simulink model "sim_tcst_2024_att_ctrl"  (R2020a)
settings: Solver=ode4  StartTime=0.0  StopTime=30.0  FixedStep=0.01  RelTol=1e-3
values from neighbouring files (symbols this model uses):
  beta0 = 2    [init_tcst_2024_att_ctrl.m]
  c1_diff_sigma_bar_w = diag([12; 12; 12])    [init_tcst_2024_att_ctrl.m]
  c1_diff_ui = diag([25; 30; 20])    [init_tcst_2024_att_ctrl.m]
  c2_diff_sigma_bar_w = diag([12; 12; 12])    [init_tcst_2024_att_ctrl.m]
  c2_diff_ui = diag([50; 50; 10])    [init_tcst_2024_att_ctrl.m]
  c3_diff_sigma_bar_w = diag([15; 15; 15])    [init_tcst_2024_att_ctrl.m]
  c3_diff_ui = diag([15; 15; 10])    [init_tcst_2024_att_ctrl.m]
  dw_aa_t = 0.2 * ones(3, 5) + ( 1.0 - 0.2 ) * rand(3, 5)    [init_tcst_2024_att_ctrl.m]
  dw_ff_t = [ 0.4 * ones(1, 5) + ( 1.0 - 0.4 ) * rand(1, 5);                      0.4 * ones(1, 5) + ( 1.0 - 0.4 ) * rand(1, 5);                      0.2 * ones(1, 5) + ( 0.6 - 0.2 ) * rand(1, 5) ]    [init_tcst_2024_att_ctrl.m]
  dw_phi_t = ( - pi / 2 ) * ones(3, 5) + ( pi / 2 - ( - pi / 2 ) ) * rand(3, 5)    [init_tcst_2024_att_ctrl.m]
  dwci_init = zeros(3,5)    [init_tcst_2024_att_ctrl.m]
  err_Ri_bar_init = zeros(3,NF)    [init_tcst_2024_att_ctrl.m]
  Fi_init = zeros(3,NF)    [init_tcst_2024_att_ctrl.m]
  h1w = diag([20.0; 20.0; 20.0])    [init_tcst_2024_att_ctrl.m]
  h2w = diag([30.0; 35.0; 35.0])    [init_tcst_2024_att_ctrl.m]
  h3w = diag([30.0; 25.0; 30.0])    [init_tcst_2024_att_ctrl.m]
  Ji = zeros(3,3,NF)    [init_tcst_2024_att_ctrl.m]
  kr1 = 10    [init_tcst_2024_att_ctrl.m]
  kr2 = 10    [init_tcst_2024_att_ctrl.m]
  kr3 = 5    [init_tcst_2024_att_ctrl.m]
  Lamd_diff_sigma_bar_w = 0.8    [init_tcst_2024_att_ctrl.m]
  Lamd_diff_ui = 0.8    [init_tcst_2024_att_ctrl.m]
  mu_d_w = 100    [init_tcst_2024_att_ctrl.m]
  pos0 = zeros(3, 1)    [init_tcst_2024_att_ctrl.m]
  PZ0 = P0(3)    [init_tcst_2024_att_ctrl.m]
  PZ1 = 10    [init_tcst_2024_att_ctrl.m]
  Qci_init = repmat([1;0;0;0],1,NF)    [init_tcst_2024_att_ctrl.m]
  Qei_init = zeros(4,NF)    [init_tcst_2024_att_ctrl.m]
  R0 = 4    [init_tcst_2024_att_ctrl.m]
  R1 = 8    [init_tcst_2024_att_ctrl.m]
  Rci_init = zeros(3,3,NF)    [init_tcst_2024_att_ctrl.m]
  Rei_init = zeros(3,3,NF)    [init_tcst_2024_att_ctrl.m]
  Ri_init = zeros(3,3,NF)    [init_tcst_2024_att_ctrl.m]
  Rx2 = 10    [init_tcst_2024_att_ctrl.m]
  Ry2 = 6    [init_tcst_2024_att_ctrl.m]
  Rz2 = 4    [init_tcst_2024_att_ctrl.m]
  T0 = 0    [init_tcst_2024_att_ctrl.m]
  T1 = tseq1    (= 10)    [init_tcst_2024_att_ctrl.m]
  T2 = tseq1 + tseq12 + tseq2    (= 30)    [init_tcst_2024_att_ctrl.m]
  ui_init = zeros(3,NF)    [init_tcst_2024_att_ctrl.m]
  V_Phi_Rei_init = zeros(3,NF)    [init_tcst_2024_att_ctrl.m]
  vel0 = zeros(3, 1)    [init_tcst_2024_att_ctrl.m]
  wci_init = zeros(3,5)    [init_tcst_2024_att_ctrl.m]
  wei_init = zeros(3,NF)    [init_tcst_2024_att_ctrl.m]
  zeta_diff_sigma_bar_w = 0.3    [init_tcst_2024_att_ctrl.m]
  zeta_diff_ui = 0.05    [init_tcst_2024_att_ctrl.m]
undefined symbols (not defined in the file or in its folder): cal_frac_squ, p_alfaw1, p_alfaw2, q_alfaw1, q_alfaw2, Qi_init, wi_init
(part 2 of 4)

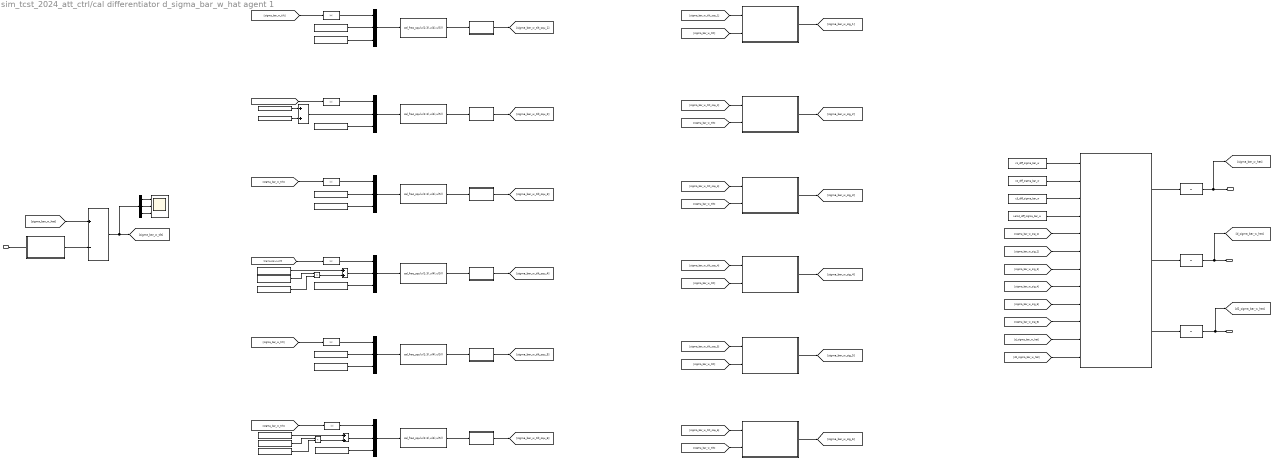
== system sim_tcst_2024_att_ctrl/cal differentiator d_sigma_bar_w_hat agent 1 ==
  x : Inport
  Abs{,1..5} (6 alike) : Abs
  Add : Sum
  Add1 : Sum
  Add2 : Sum
  Add3 : Sum  Inputs=+-
  Constant : Constant  Value=0
  Constant{97,100,105,107,109} (5 alike) : Constant
  Constant{98..99,101,108,110..111} (6 alike) : Constant  Value=3
  Constant102 : Constant  Value=2
  Constant103 : Constant  Value=c1_diff_sigma_bar_w
  Constant104 : Constant  Value=c2_diff_sigma_bar_w
  Constant106 : Constant  Value=c3_diff_sigma_bar_w
  Constant112 : Constant  Value=2
  Constant113 : Constant  Value=Lamd_diff_sigma_bar_w
  Constant161 : Constant  Value=zeta_diff_sigma_bar_w
  Constant162 : Constant  Value=zeta_diff_sigma_bar_w
  Constant163 : Constant  Value=zeta_diff_sigma_bar_w
  Demux2 : Demux  Outputs=3
  Integrator2 : Integrator  InitialCondition=zeros(3,1)
  Integrator3 : Integrator  InitialCondition=zeros(3,1)
  Integrator4 : Integrator  InitialCondition=zeros(3,1)
  Interpreted MATLAB Function{,20..24} (6 alike) : MATLABFcn  MATLABFcn=cal_frac_squ(u(1:3),u(4),u(5))
  Mux{19..24} (6 alike) : Mux  Inputs=3
  Product : Product
  Product1 : Product
  cal differentiator : MATLAB Function  TreatAsAtomicUnit=on
  cal sig : MATLAB Function  TreatAsAtomicUnit=on
  cal sig1 : MATLAB Function  TreatAsAtomicUnit=on
  cal sig2 : MATLAB Function  TreatAsAtomicUnit=on
  cal sig3 : MATLAB Function  TreatAsAtomicUnit=on
  cal sig4 : MATLAB Function  TreatAsAtomicUnit=on
  cal sig5 : MATLAB Function  TreatAsAtomicUnit=on
  choose sigma_bar_w : MATLAB Function  TreatAsAtomicUnit=on
  sigma_bar_w_tilt : Scope  NumInputPorts=3
  trans to column20 : MATLAB Function  TreatAsAtomicUnit=on
  trans to column21 : MATLAB Function  TreatAsAtomicUnit=on
  trans to column22 : MATLAB Function  TreatAsAtomicUnit=on
  trans to column23 : MATLAB Function  TreatAsAtomicUnit=on
  trans to column24 : MATLAB Function  TreatAsAtomicUnit=on
  trans to column25 : MATLAB Function  TreatAsAtomicUnit=on
  Out1 : Outport
  Out2 : Outport  Port=2
  Out3 : Outport  Port=3
  wires:
  Abs/1 -> Mux22/1
  [sigma_bar_w_tilt] -> cal sig/2(y)
  cal sig1/1(z) -> [sigma_bar_w_sig_2]
  [d2_sigma_bar_w_hat] -> cal differentiator/12(d2_sigma_bar_v_hat)
  trans to column23/1(y) -> [sigma_bar_w_tilt_squ_3]
  Add/1 -> Mux21/2
  Demux2/1 -> sigma_bar_w_tilt/1
  [sigma_bar_w_tilt] -> cal sig4/2(y)
  Product1/1 -> Add2/2
  Add2/1 -> Mux19/2
  [d_sigma_bar_w_hat] -> cal differentiator/11("d_sigma_bar_v_hat ")
  [sigma_bar_w_sig_3] -> cal differentiator/7(sigma_bar_v_sig_3)
  trans to column24/1(y) -> [sigma_bar_w_tilt_squ_4]
  Constant107/1 -> Mux21/3
  [sigma_bar_w_sig_5] -> cal differentiator/9(sigma_bar_v_sig_5)
  Constant97/1 -> Mux22/3
  cal sig/1(z) -> [sigma_bar_w_sig_1]
  trans to column22/1(y) -> [sigma_bar_w_tilt_squ_1]
  [sigma_bar_w_tilt_squ_3] -> cal sig2/1(x)
  [sigma_bar_w_tilt] -> Abs3/1
  Interpreted MATLAB Function24/1 -> trans to column25/1(x)
  [sigma_bar_w_sig_1] -> cal differentiator/5(sigma_bar_v_sig_1)
  cal differentiator/1(d_sigma_bar_v_hat) -> Integrator2/1
  Constant110/1 -> Mux24/3
  cal sig5/1(z) -> [sigma_bar_w_sig_5]
  [sigma_bar_w_tilt] -> Abs4/1
  Demux2/3 -> sigma_bar_w_tilt/3
  cal sig2/1(z) -> [sigma_bar_w_sig_3]
  Constant112/1 -> Product/1
  Constant/1 -> Mux22/2
  cal differentiator/3(d_d2sigma_bar_v_hat) -> Integrator4/1
  Abs3/1 -> Mux24/1
  trans to column21/1(y) -> [sigma_bar_w_tilt_squ_2]
  Constant99/1 -> Add2/1
  Constant103/1 -> cal differentiator/1(c1)
  Mux19/1 -> Interpreted MATLAB Function24/1
  [sigma_bar_w_tilt_squ_6] -> cal sig3/1(x)
  Constant106/1 -> cal differentiator/3(c3)
  [sigma_bar_w_tilt] -> Abs2/1
  [sigma_bar_w_tilt_squ_2] -> cal sig1/1(x)
  Constant162/1 -> Product/2
  Product/1 -> Add1/2
  [sigma_bar_w_sig_4] -> cal differentiator/8(sigma_bar_v_sig_4)
  [sigma_bar_w_hat] -> Add3/1
  Constant102/1 -> Mux20/2
  Add3/1 -> Demux2/1, [sigma_bar_w_tilt]
  cal differentiator/2(d_dsigma_bar_v_hat) -> Integrator3/1
  [sigma_bar_w_tilt] -> Abs5/1
  [sigma_bar_w_tilt] -> cal sig2/2(y)
  [sigma_bar_w_sig_6] -> cal differentiator/10(sigma_bar_v_sig_6)
  trans to column20/1(y) -> [sigma_bar_w_tilt_squ_5]
  Constant104/1 -> cal differentiator/2(c2)
  Constant101/1 -> Mux20/3
  Mux22/1 -> Interpreted MATLAB Function/1
  Constant163/1 -> Product1/2
  Abs2/1 -> Mux23/1
  Interpreted MATLAB Function21/1 -> trans to column21/1(x)
  Interpreted MATLAB Function23/1 -> trans to column24/1(x)
  Mux23/1 -> Interpreted MATLAB Function22/1
  cal sig3/1(z) -> [sigma_bar_w_sig_6]
  Abs4/1 -> Mux19/1
  trans to column25/1(y) -> [sigma_bar_w_tilt_squ_6]
  Constant113/1 -> cal differentiator/4(chi_t)
  choose sigma_bar_w/1(y) -> Add3/2
  Interpreted MATLAB Function/1 -> trans to column22/1(x)
  Interpreted MATLAB Function20/1 -> trans to column20/1(x)
  Constant108/1 -> Mux23/3
  [sigma_bar_w_sig_2] -> cal differentiator/6(sigma_bar_v_sig_2)
  [sigma_bar_w_tilt] -> cal sig1/2(y)
  [sigma_bar_w_tilt_squ_1] -> cal sig/1(x)
  Constant100/1 -> Product1/1
  Abs1/1 -> Mux21/1
  Demux2/2 -> sigma_bar_w_tilt/2
  Integrator4/1 -> [d2_sigma_bar_w_hat], Out3/1
  [sigma_bar_w_tilt_squ_4] -> cal sig4/1(x)
  Abs5/1 -> Mux20/1
  Constant98/1 -> Mux19/3
  Constant111/1 -> Add1/1
  [sigma_bar_w_tilt] -> cal sig5/2(y)
  Constant109/1 -> Mux23/2
  [sigma_bar_w_tilt] -> Abs/1
  Mux24/1 -> Interpreted MATLAB Function23/1
  [sigma_bar_w_tilt] -> Abs1/1
  [sigma_bar_w_tilt_squ_5] -> cal sig5/1(x)
  Add1/1 -> Mux24/2
  cal sig4/1(z) -> [sigma_bar_w_sig_4]
  Constant161/1 -> Add/2
  [sigma_bar_w_tilt] -> cal sig3/2(y)
  Mux21/1 -> Interpreted MATLAB Function21/1
  Interpreted MATLAB Function22/1 -> trans to column23/1(x)
  Mux20/1 -> Interpreted MATLAB Function20/1
  x/1 -> choose sigma_bar_w/1(x)
  Constant105/1 -> Add/1
  Integrator2/1 -> [sigma_bar_w_hat], Out1/1
  Integrator3/1 -> [d_sigma_bar_w_hat], Out2/1

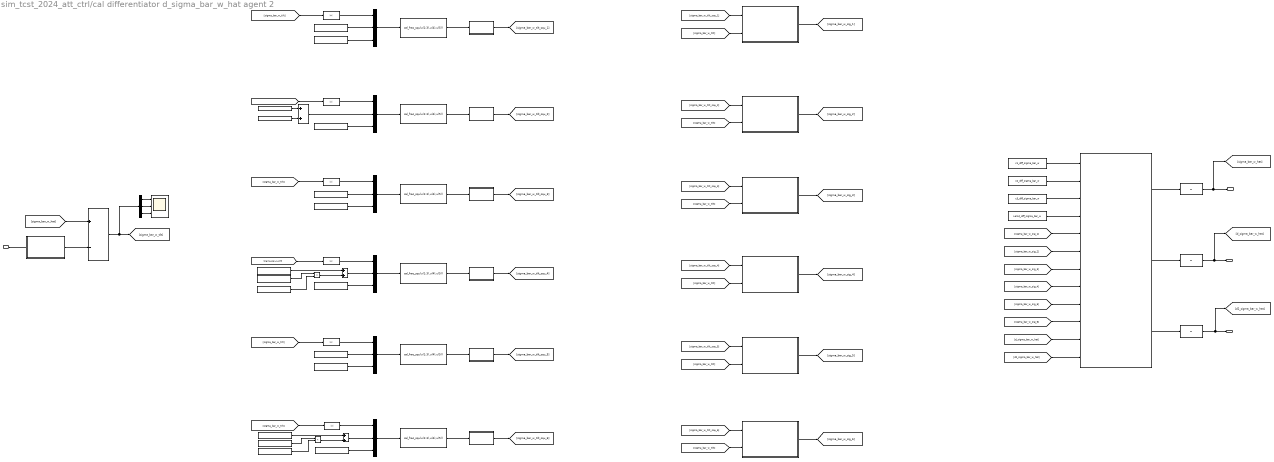
== system sim_tcst_2024_att_ctrl/cal differentiator d_sigma_bar_w_hat agent 2 ==
  x : Inport
  Abs{,1..5} (6 alike) : Abs
  Add : Sum
  Add1 : Sum
  Add2 : Sum
  Add3 : Sum  Inputs=+-
  Constant : Constant  Value=0
  Constant{97,100,105,107,109} (5 alike) : Constant
  Constant{98..99,101,108,110..111} (6 alike) : Constant  Value=3
  Constant102 : Constant  Value=2
  Constant103 : Constant  Value=c1_diff_sigma_bar_w
  Constant104 : Constant  Value=c2_diff_sigma_bar_w
  Constant106 : Constant  Value=c3_diff_sigma_bar_w
  Constant112 : Constant  Value=2
  Constant113 : Constant  Value=Lamd_diff_sigma_bar_w
  Constant161 : Constant  Value=zeta_diff_sigma_bar_w
  Constant162 : Constant  Value=zeta_diff_sigma_bar_w
  Constant163 : Constant  Value=zeta_diff_sigma_bar_w
  Demux2 : Demux  Outputs=3
  Integrator2 : Integrator  InitialCondition=zeros(3,1)
  Integrator3 : Integrator  InitialCondition=zeros(3,1)
  Integrator4 : Integrator  InitialCondition=zeros(3,1)
  Interpreted MATLAB Function{,20..24} (6 alike) : MATLABFcn  MATLABFcn=cal_frac_squ(u(1:3),u(4),u(5))
  Mux{19..24} (6 alike) : Mux  Inputs=3
  Product : Product
  Product1 : Product
  cal differentiator : MATLAB Function  TreatAsAtomicUnit=on
  cal sig : MATLAB Function  TreatAsAtomicUnit=on
  cal sig1 : MATLAB Function  TreatAsAtomicUnit=on
  cal sig2 : MATLAB Function  TreatAsAtomicUnit=on
  cal sig3 : MATLAB Function  TreatAsAtomicUnit=on
  cal sig4 : MATLAB Function  TreatAsAtomicUnit=on
  cal sig5 : MATLAB Function  TreatAsAtomicUnit=on
  choose sigma_bar_w : MATLAB Function  TreatAsAtomicUnit=on
  sigma_bar_w_tilt : Scope  NumInputPorts=3
  trans to column20 : MATLAB Function  TreatAsAtomicUnit=on
  trans to column21 : MATLAB Function  TreatAsAtomicUnit=on
  trans to column22 : MATLAB Function  TreatAsAtomicUnit=on
  trans to column23 : MATLAB Function  TreatAsAtomicUnit=on
  trans to column24 : MATLAB Function  TreatAsAtomicUnit=on
  trans to column25 : MATLAB Function  TreatAsAtomicUnit=on
  Out1 : Outport
  Out2 : Outport  Port=2
  Out3 : Outport  Port=3
  wires:
  Abs/1 -> Mux22/1
  [sigma_bar_w_tilt] -> cal sig/2(y)
  cal sig1/1(z) -> [sigma_bar_w_sig_2]
  [d2_sigma_bar_w_hat] -> cal differentiator/12(d2_sigma_bar_v_hat)
  trans to column23/1(y) -> [sigma_bar_w_tilt_squ_3]
  Add/1 -> Mux21/2
  Demux2/1 -> sigma_bar_w_tilt/1
  [sigma_bar_w_tilt] -> cal sig4/2(y)
  Product1/1 -> Add2/2
  Add2/1 -> Mux19/2
  [d_sigma_bar_w_hat] -> cal differentiator/11("d_sigma_bar_v_hat ")
  [sigma_bar_w_sig_3] -> cal differentiator/7(sigma_bar_v_sig_3)
  trans to column24/1(y) -> [sigma_bar_w_tilt_squ_4]
  Constant107/1 -> Mux21/3
  [sigma_bar_w_sig_5] -> cal differentiator/9(sigma_bar_v_sig_5)
  Constant97/1 -> Mux22/3
  cal sig/1(z) -> [sigma_bar_w_sig_1]
  trans to column22/1(y) -> [sigma_bar_w_tilt_squ_1]
  [sigma_bar_w_tilt_squ_3] -> cal sig2/1(x)
  [sigma_bar_w_tilt] -> Abs3/1
  Interpreted MATLAB Function24/1 -> trans to column25/1(x)
  [sigma_bar_w_sig_1] -> cal differentiator/5(sigma_bar_v_sig_1)
  cal differentiator/1(d_sigma_bar_v_hat) -> Integrator2/1
  Constant110/1 -> Mux24/3
  cal sig5/1(z) -> [sigma_bar_w_sig_5]
  [sigma_bar_w_tilt] -> Abs4/1
  Demux2/3 -> sigma_bar_w_tilt/3
  cal sig2/1(z) -> [sigma_bar_w_sig_3]
  Constant112/1 -> Product/1
  Constant/1 -> Mux22/2
  cal differentiator/3(d_d2sigma_bar_v_hat) -> Integrator4/1
  Abs3/1 -> Mux24/1
  trans to column21/1(y) -> [sigma_bar_w_tilt_squ_2]
  Constant99/1 -> Add2/1
  Constant103/1 -> cal differentiator/1(c1)
  Mux19/1 -> Interpreted MATLAB Function24/1
  [sigma_bar_w_tilt_squ_6] -> cal sig3/1(x)
  Constant106/1 -> cal differentiator/3(c3)
  [sigma_bar_w_tilt] -> Abs2/1
  [sigma_bar_w_tilt_squ_2] -> cal sig1/1(x)
  Constant162/1 -> Product/2
  Product/1 -> Add1/2
  [sigma_bar_w_sig_4] -> cal differentiator/8(sigma_bar_v_sig_4)
  [sigma_bar_w_hat] -> Add3/1
  Constant102/1 -> Mux20/2
  Add3/1 -> Demux2/1, [sigma_bar_w_tilt]
  cal differentiator/2(d_dsigma_bar_v_hat) -> Integrator3/1
  [sigma_bar_w_tilt] -> Abs5/1
  [sigma_bar_w_tilt] -> cal sig2/2(y)
  [sigma_bar_w_sig_6] -> cal differentiator/10(sigma_bar_v_sig_6)
  trans to column20/1(y) -> [sigma_bar_w_tilt_squ_5]
  Constant104/1 -> cal differentiator/2(c2)
  Constant101/1 -> Mux20/3
  Mux22/1 -> Interpreted MATLAB Function/1
  Constant163/1 -> Product1/2
  Abs2/1 -> Mux23/1
  Interpreted MATLAB Function21/1 -> trans to column21/1(x)
  Interpreted MATLAB Function23/1 -> trans to column24/1(x)
  Mux23/1 -> Interpreted MATLAB Function22/1
  cal sig3/1(z) -> [sigma_bar_w_sig_6]
  Abs4/1 -> Mux19/1
  trans to column25/1(y) -> [sigma_bar_w_tilt_squ_6]
  Constant113/1 -> cal differentiator/4(chi_t)
  choose sigma_bar_w/1(y) -> Add3/2
  Interpreted MATLAB Function/1 -> trans to column22/1(x)
  Interpreted MATLAB Function20/1 -> trans to column20/1(x)
  Constant108/1 -> Mux23/3
  [sigma_bar_w_sig_2] -> cal differentiator/6(sigma_bar_v_sig_2)
  [sigma_bar_w_tilt] -> cal sig1/2(y)
  [sigma_bar_w_tilt_squ_1] -> cal sig/1(x)
  Constant100/1 -> Product1/1
  Abs1/1 -> Mux21/1
  Demux2/2 -> sigma_bar_w_tilt/2
  Integrator4/1 -> [d2_sigma_bar_w_hat], Out3/1
  [sigma_bar_w_tilt_squ_4] -> cal sig4/1(x)
  Abs5/1 -> Mux20/1
  Constant98/1 -> Mux19/3
  Constant111/1 -> Add1/1
  [sigma_bar_w_tilt] -> cal sig5/2(y)
  Constant109/1 -> Mux23/2
  [sigma_bar_w_tilt] -> Abs/1
  Mux24/1 -> Interpreted MATLAB Function23/1
  [sigma_bar_w_tilt] -> Abs1/1
  [sigma_bar_w_tilt_squ_5] -> cal sig5/1(x)
  Add1/1 -> Mux24/2
  cal sig4/1(z) -> [sigma_bar_w_sig_4]
  Constant161/1 -> Add/2
  [sigma_bar_w_tilt] -> cal sig3/2(y)
  Mux21/1 -> Interpreted MATLAB Function21/1
  Interpreted MATLAB Function22/1 -> trans to column23/1(x)
  Mux20/1 -> Interpreted MATLAB Function20/1
  x/1 -> choose sigma_bar_w/1(x)
  Constant105/1 -> Add/1
  Integrator2/1 -> [sigma_bar_w_hat], Out1/1
  Integrator3/1 -> [d_sigma_bar_w_hat], Out2/1

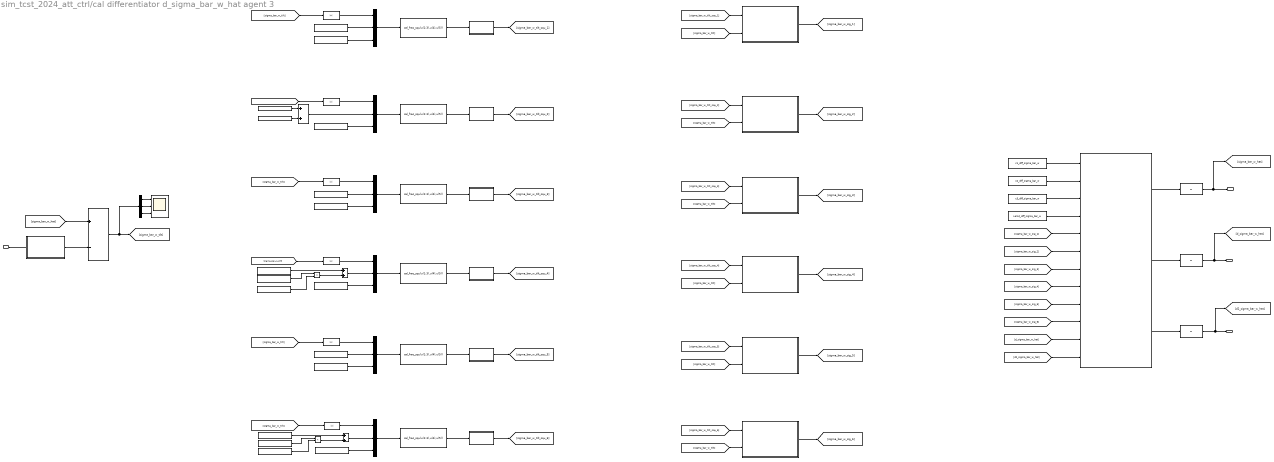
== system sim_tcst_2024_att_ctrl/cal differentiator d_sigma_bar_w_hat agent 3 ==
  x : Inport
  Abs{,1..5} (6 alike) : Abs
  Add : Sum
  Add1 : Sum
  Add2 : Sum
  Add3 : Sum  Inputs=+-
  Constant : Constant  Value=0
  Constant{97,100,105,107,109} (5 alike) : Constant
  Constant{98..99,101,108,110..111} (6 alike) : Constant  Value=3
  Constant102 : Constant  Value=2
  Constant103 : Constant  Value=c1_diff_sigma_bar_w
  Constant104 : Constant  Value=c2_diff_sigma_bar_w
  Constant106 : Constant  Value=c3_diff_sigma_bar_w
  Constant112 : Constant  Value=2
  Constant113 : Constant  Value=Lamd_diff_sigma_bar_w
  Constant161 : Constant  Value=zeta_diff_sigma_bar_w
  Constant162 : Constant  Value=zeta_diff_sigma_bar_w
  Constant163 : Constant  Value=zeta_diff_sigma_bar_w
  Demux2 : Demux  Outputs=3
  Integrator2 : Integrator  InitialCondition=zeros(3,1)
  Integrator3 : Integrator  InitialCondition=zeros(3,1)
  Integrator4 : Integrator  InitialCondition=zeros(3,1)
  Interpreted MATLAB Function{,20..24} (6 alike) : MATLABFcn  MATLABFcn=cal_frac_squ(u(1:3),u(4),u(5))
  Mux{19..24} (6 alike) : Mux  Inputs=3
  Product : Product
  Product1 : Product
  cal differentiator : MATLAB Function  TreatAsAtomicUnit=on
  cal sig : MATLAB Function  TreatAsAtomicUnit=on
  cal sig1 : MATLAB Function  TreatAsAtomicUnit=on
  cal sig2 : MATLAB Function  TreatAsAtomicUnit=on
  cal sig3 : MATLAB Function  TreatAsAtomicUnit=on
  cal sig4 : MATLAB Function  TreatAsAtomicUnit=on
  cal sig5 : MATLAB Function  TreatAsAtomicUnit=on
  choose sigma_bar_w : MATLAB Function  TreatAsAtomicUnit=on
  sigma_bar_w_tilt : Scope  NumInputPorts=3
  trans to column20 : MATLAB Function  TreatAsAtomicUnit=on
  trans to column21 : MATLAB Function  TreatAsAtomicUnit=on
  trans to column22 : MATLAB Function  TreatAsAtomicUnit=on
  trans to column23 : MATLAB Function  TreatAsAtomicUnit=on
  trans to column24 : MATLAB Function  TreatAsAtomicUnit=on
  trans to column25 : MATLAB Function  TreatAsAtomicUnit=on
  Out1 : Outport
  Out2 : Outport  Port=2
  Out3 : Outport  Port=3
  wires:
  Abs/1 -> Mux22/1
  [sigma_bar_w_tilt] -> cal sig/2(y)
  cal sig1/1(z) -> [sigma_bar_w_sig_2]
  [d2_sigma_bar_w_hat] -> cal differentiator/12(d2_sigma_bar_v_hat)
  trans to column23/1(y) -> [sigma_bar_w_tilt_squ_3]
  Add/1 -> Mux21/2
  Demux2/1 -> sigma_bar_w_tilt/1
  [sigma_bar_w_tilt] -> cal sig4/2(y)
  Product1/1 -> Add2/2
  Add2/1 -> Mux19/2
  [d_sigma_bar_w_hat] -> cal differentiator/11("d_sigma_bar_v_hat ")
  [sigma_bar_w_sig_3] -> cal differentiator/7(sigma_bar_v_sig_3)
  trans to column24/1(y) -> [sigma_bar_w_tilt_squ_4]
  Constant107/1 -> Mux21/3
  [sigma_bar_w_sig_5] -> cal differentiator/9(sigma_bar_v_sig_5)
  Constant97/1 -> Mux22/3
  cal sig/1(z) -> [sigma_bar_w_sig_1]
  trans to column22/1(y) -> [sigma_bar_w_tilt_squ_1]
  [sigma_bar_w_tilt_squ_3] -> cal sig2/1(x)
  [sigma_bar_w_tilt] -> Abs3/1
  Interpreted MATLAB Function24/1 -> trans to column25/1(x)
  [sigma_bar_w_sig_1] -> cal differentiator/5(sigma_bar_v_sig_1)
  cal differentiator/1(d_sigma_bar_v_hat) -> Integrator2/1
  Constant110/1 -> Mux24/3
  cal sig5/1(z) -> [sigma_bar_w_sig_5]
  [sigma_bar_w_tilt] -> Abs4/1
  Demux2/3 -> sigma_bar_w_tilt/3
  cal sig2/1(z) -> [sigma_bar_w_sig_3]
  Constant112/1 -> Product/1
  Constant/1 -> Mux22/2
  cal differentiator/3(d_d2sigma_bar_v_hat) -> Integrator4/1
  Abs3/1 -> Mux24/1
  trans to column21/1(y) -> [sigma_bar_w_tilt_squ_2]
  Constant99/1 -> Add2/1
  Constant103/1 -> cal differentiator/1(c1)
  Mux19/1 -> Interpreted MATLAB Function24/1
  [sigma_bar_w_tilt_squ_6] -> cal sig3/1(x)
  Constant106/1 -> cal differentiator/3(c3)
  [sigma_bar_w_tilt] -> Abs2/1
  [sigma_bar_w_tilt_squ_2] -> cal sig1/1(x)
  Constant162/1 -> Product/2
  Product/1 -> Add1/2
  [sigma_bar_w_sig_4] -> cal differentiator/8(sigma_bar_v_sig_4)
  [sigma_bar_w_hat] -> Add3/1
  Constant102/1 -> Mux20/2
  Add3/1 -> Demux2/1, [sigma_bar_w_tilt]
  cal differentiator/2(d_dsigma_bar_v_hat) -> Integrator3/1
  [sigma_bar_w_tilt] -> Abs5/1
  [sigma_bar_w_tilt] -> cal sig2/2(y)
  [sigma_bar_w_sig_6] -> cal differentiator/10(sigma_bar_v_sig_6)
  trans to column20/1(y) -> [sigma_bar_w_tilt_squ_5]
  Constant104/1 -> cal differentiator/2(c2)
  Constant101/1 -> Mux20/3
  Mux22/1 -> Interpreted MATLAB Function/1
  Constant163/1 -> Product1/2
  Abs2/1 -> Mux23/1
  Interpreted MATLAB Function21/1 -> trans to column21/1(x)
  Interpreted MATLAB Function23/1 -> trans to column24/1(x)
  Mux23/1 -> Interpreted MATLAB Function22/1
  cal sig3/1(z) -> [sigma_bar_w_sig_6]
  Abs4/1 -> Mux19/1
  trans to column25/1(y) -> [sigma_bar_w_tilt_squ_6]
  Constant113/1 -> cal differentiator/4(chi_t)
  choose sigma_bar_w/1(y) -> Add3/2
  Interpreted MATLAB Function/1 -> trans to column22/1(x)
  Interpreted MATLAB Function20/1 -> trans to column20/1(x)
  Constant108/1 -> Mux23/3
  [sigma_bar_w_sig_2] -> cal differentiator/6(sigma_bar_v_sig_2)
  [sigma_bar_w_tilt] -> cal sig1/2(y)
  [sigma_bar_w_tilt_squ_1] -> cal sig/1(x)
  Constant100/1 -> Product1/1
  Abs1/1 -> Mux21/1
  Demux2/2 -> sigma_bar_w_tilt/2
  Integrator4/1 -> [d2_sigma_bar_w_hat], Out3/1
  [sigma_bar_w_tilt_squ_4] -> cal sig4/1(x)
  Abs5/1 -> Mux20/1
  Constant98/1 -> Mux19/3
  Constant111/1 -> Add1/1
  [sigma_bar_w_tilt] -> cal sig5/2(y)
  Constant109/1 -> Mux23/2
  [sigma_bar_w_tilt] -> Abs/1
  Mux24/1 -> Interpreted MATLAB Function23/1
  [sigma_bar_w_tilt] -> Abs1/1
  [sigma_bar_w_tilt_squ_5] -> cal sig5/1(x)
  Add1/1 -> Mux24/2
  cal sig4/1(z) -> [sigma_bar_w_sig_4]
  Constant161/1 -> Add/2
  [sigma_bar_w_tilt] -> cal sig3/2(y)
  Mux21/1 -> Interpreted MATLAB Function21/1
  Interpreted MATLAB Function22/1 -> trans to column23/1(x)
  Mux20/1 -> Interpreted MATLAB Function20/1
  x/1 -> choose sigma_bar_w/1(x)
  Constant105/1 -> Add/1
  Integrator2/1 -> [sigma_bar_w_hat], Out1/1
  Integrator3/1 -> [d_sigma_bar_w_hat], Out2/1

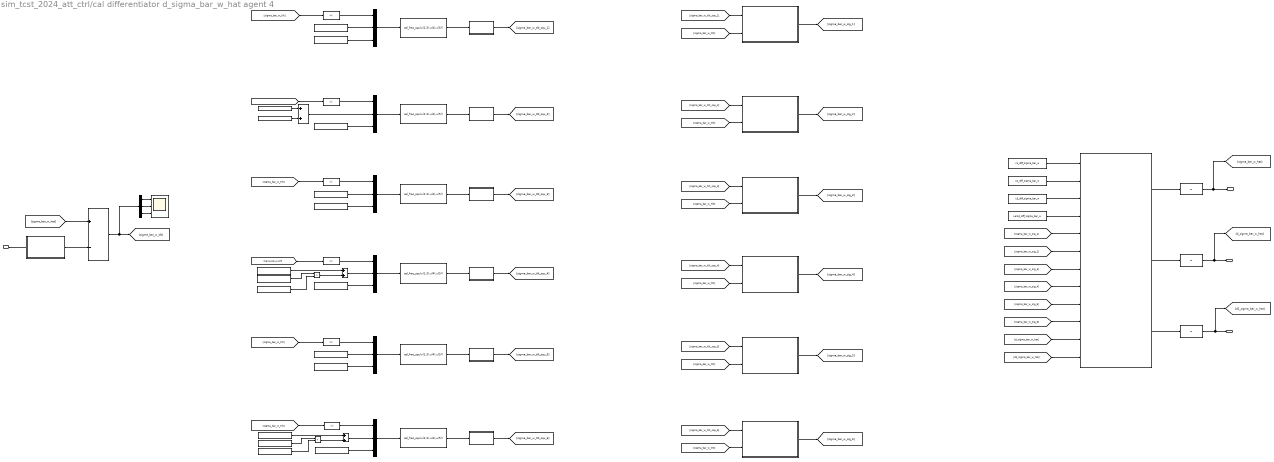
== system sim_tcst_2024_att_ctrl/cal differentiator d_sigma_bar_w_hat agent 4 ==
  x : Inport
  Abs{,1..5} (6 alike) : Abs
  Add : Sum
  Add1 : Sum
  Add2 : Sum
  Add3 : Sum  Inputs=+-
  Constant : Constant  Value=0
  Constant{97,100,105,107,109} (5 alike) : Constant
  Constant{98..99,101,108,110..111} (6 alike) : Constant  Value=3
  Constant102 : Constant  Value=2
  Constant103 : Constant  Value=c1_diff_sigma_bar_w
  Constant104 : Constant  Value=c2_diff_sigma_bar_w
  Constant106 : Constant  Value=c3_diff_sigma_bar_w
  Constant112 : Constant  Value=2
  Constant113 : Constant  Value=Lamd_diff_sigma_bar_w
  Constant161 : Constant  Value=zeta_diff_sigma_bar_w
  Constant162 : Constant  Value=zeta_diff_sigma_bar_w
  Constant163 : Constant  Value=zeta_diff_sigma_bar_w
  Demux2 : Demux  Outputs=3
  Integrator2 : Integrator  InitialCondition=zeros(3,1)
  Integrator3 : Integrator  InitialCondition=zeros(3,1)
  Integrator4 : Integrator  InitialCondition=zeros(3,1)
  Interpreted MATLAB Function{,20..24} (6 alike) : MATLABFcn  MATLABFcn=cal_frac_squ(u(1:3),u(4),u(5))
  Mux{19..24} (6 alike) : Mux  Inputs=3
  Product : Product
  Product1 : Product
  cal differentiator : MATLAB Function  TreatAsAtomicUnit=on
  cal sig : MATLAB Function  TreatAsAtomicUnit=on
  cal sig1 : MATLAB Function  TreatAsAtomicUnit=on
  cal sig2 : MATLAB Function  TreatAsAtomicUnit=on
  cal sig3 : MATLAB Function  TreatAsAtomicUnit=on
  cal sig4 : MATLAB Function  TreatAsAtomicUnit=on
  cal sig5 : MATLAB Function  TreatAsAtomicUnit=on
  choose sigma_bar_w : MATLAB Function  TreatAsAtomicUnit=on
  sigma_bar_w_tilt : Scope  NumInputPorts=3
  trans to column20 : MATLAB Function  TreatAsAtomicUnit=on
  trans to column21 : MATLAB Function  TreatAsAtomicUnit=on
  trans to column22 : MATLAB Function  TreatAsAtomicUnit=on
  trans to column23 : MATLAB Function  TreatAsAtomicUnit=on
  trans to column24 : MATLAB Function  TreatAsAtomicUnit=on
  trans to column25 : MATLAB Function  TreatAsAtomicUnit=on
  Out1 : Outport
  Out2 : Outport  Port=2
  Out3 : Outport  Port=3
  wires:
  Abs/1 -> Mux22/1
  [sigma_bar_w_tilt] -> cal sig/2(y)
  cal sig1/1(z) -> [sigma_bar_w_sig_2]
  [d2_sigma_bar_w_hat] -> cal differentiator/12(d2_sigma_bar_v_hat)
  trans to column23/1(y) -> [sigma_bar_w_tilt_squ_3]
  Add/1 -> Mux21/2
  Demux2/1 -> sigma_bar_w_tilt/1
  [sigma_bar_w_tilt] -> cal sig4/2(y)
  Product1/1 -> Add2/2
  Add2/1 -> Mux19/2
  [d_sigma_bar_w_hat] -> cal differentiator/11("d_sigma_bar_v_hat ")
  [sigma_bar_w_sig_3] -> cal differentiator/7(sigma_bar_v_sig_3)
  trans to column24/1(y) -> [sigma_bar_w_tilt_squ_4]
  Constant107/1 -> Mux21/3
  [sigma_bar_w_sig_5] -> cal differentiator/9(sigma_bar_v_sig_5)
  Constant97/1 -> Mux22/3
  cal sig/1(z) -> [sigma_bar_w_sig_1]
  trans to column22/1(y) -> [sigma_bar_w_tilt_squ_1]
  [sigma_bar_w_tilt_squ_3] -> cal sig2/1(x)
  [sigma_bar_w_tilt] -> Abs3/1
  Interpreted MATLAB Function24/1 -> trans to column25/1(x)
  [sigma_bar_w_sig_1] -> cal differentiator/5(sigma_bar_v_sig_1)
  cal differentiator/1(d_sigma_bar_v_hat) -> Integrator2/1
  Constant110/1 -> Mux24/3
  cal sig5/1(z) -> [sigma_bar_w_sig_5]
  [sigma_bar_w_tilt] -> Abs4/1
  Demux2/3 -> sigma_bar_w_tilt/3
  cal sig2/1(z) -> [sigma_bar_w_sig_3]
  Constant112/1 -> Product/1
  Constant/1 -> Mux22/2
  cal differentiator/3(d_d2sigma_bar_v_hat) -> Integrator4/1
  Abs3/1 -> Mux24/1
  trans to column21/1(y) -> [sigma_bar_w_tilt_squ_2]
  Constant99/1 -> Add2/1
  Constant103/1 -> cal differentiator/1(c1)
  Mux19/1 -> Interpreted MATLAB Function24/1
  [sigma_bar_w_tilt_squ_6] -> cal sig3/1(x)
  Constant106/1 -> cal differentiator/3(c3)
  [sigma_bar_w_tilt] -> Abs2/1
  [sigma_bar_w_tilt_squ_2] -> cal sig1/1(x)
  Constant162/1 -> Product/2
  Product/1 -> Add1/2
  [sigma_bar_w_sig_4] -> cal differentiator/8(sigma_bar_v_sig_4)
  [sigma_bar_w_hat] -> Add3/1
  Constant102/1 -> Mux20/2
  Add3/1 -> Demux2/1, [sigma_bar_w_tilt]
  cal differentiator/2(d_dsigma_bar_v_hat) -> Integrator3/1
  [sigma_bar_w_tilt] -> Abs5/1
  [sigma_bar_w_tilt] -> cal sig2/2(y)
  [sigma_bar_w_sig_6] -> cal differentiator/10(sigma_bar_v_sig_6)
  trans to column20/1(y) -> [sigma_bar_w_tilt_squ_5]
  Constant104/1 -> cal differentiator/2(c2)
  Constant101/1 -> Mux20/3
  Mux22/1 -> Interpreted MATLAB Function/1
  Constant163/1 -> Product1/2
  Abs2/1 -> Mux23/1
  Interpreted MATLAB Function21/1 -> trans to column21/1(x)
  Interpreted MATLAB Function23/1 -> trans to column24/1(x)
  Mux23/1 -> Interpreted MATLAB Function22/1
  cal sig3/1(z) -> [sigma_bar_w_sig_6]
  Abs4/1 -> Mux19/1
  trans to column25/1(y) -> [sigma_bar_w_tilt_squ_6]
  Constant113/1 -> cal differentiator/4(chi_t)
  choose sigma_bar_w/1(y) -> Add3/2
  Interpreted MATLAB Function/1 -> trans to column22/1(x)
  Interpreted MATLAB Function20/1 -> trans to column20/1(x)
  Constant108/1 -> Mux23/3
  [sigma_bar_w_sig_2] -> cal differentiator/6(sigma_bar_v_sig_2)
  [sigma_bar_w_tilt] -> cal sig1/2(y)
  [sigma_bar_w_tilt_squ_1] -> cal sig/1(x)
  Constant100/1 -> Product1/1
  Abs1/1 -> Mux21/1
  Demux2/2 -> sigma_bar_w_tilt/2
  Integrator4/1 -> [d2_sigma_bar_w_hat], Out3/1
  [sigma_bar_w_tilt_squ_4] -> cal sig4/1(x)
  Abs5/1 -> Mux20/1
  Constant98/1 -> Mux19/3
  Constant111/1 -> Add1/1
  [sigma_bar_w_tilt] -> cal sig5/2(y)
  Constant109/1 -> Mux23/2
  [sigma_bar_w_tilt] -> Abs/1
  Mux24/1 -> Interpreted MATLAB Function23/1
  [sigma_bar_w_tilt] -> Abs1/1
  [sigma_bar_w_tilt_squ_5] -> cal sig5/1(x)
  Add1/1 -> Mux24/2
  cal sig4/1(z) -> [sigma_bar_w_sig_4]
  Constant161/1 -> Add/2
  [sigma_bar_w_tilt] -> cal sig3/2(y)
  Mux21/1 -> Interpreted MATLAB Function21/1
  Interpreted MATLAB Function22/1 -> trans to column23/1(x)
  Mux20/1 -> Interpreted MATLAB Function20/1
  x/1 -> choose sigma_bar_w/1(x)
  Constant105/1 -> Add/1
  Integrator2/1 -> [sigma_bar_w_hat], Out1/1
  Integrator3/1 -> [d_sigma_bar_w_hat], Out2/1

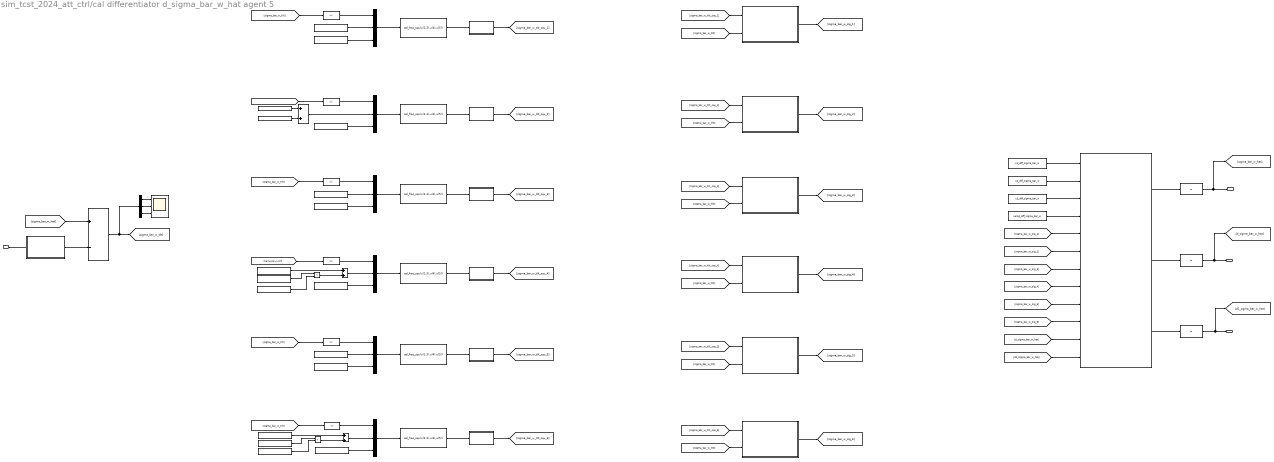
== system sim_tcst_2024_att_ctrl/cal differentiator d_sigma_bar_w_hat agent 5 ==
  x : Inport
  Abs{,1..5} (6 alike) : Abs
  Add : Sum
  Add1 : Sum
  Add2 : Sum
  Add3 : Sum  Inputs=+-
  Constant : Constant  Value=0
  Constant{97,100,105,107,109} (5 alike) : Constant
  Constant{98..99,101,108,110..111} (6 alike) : Constant  Value=3
  Constant102 : Constant  Value=2
  Constant103 : Constant  Value=c1_diff_sigma_bar_w
  Constant104 : Constant  Value=c2_diff_sigma_bar_w
  Constant106 : Constant  Value=c3_diff_sigma_bar_w
  Constant112 : Constant  Value=2
  Constant113 : Constant  Value=Lamd_diff_sigma_bar_w
  Constant161 : Constant  Value=zeta_diff_sigma_bar_w
  Constant162 : Constant  Value=zeta_diff_sigma_bar_w
  Constant163 : Constant  Value=zeta_diff_sigma_bar_w
  Demux2 : Demux  Outputs=3
  Integrator2 : Integrator  InitialCondition=zeros(3,1)
  Integrator3 : Integrator  InitialCondition=zeros(3,1)
  Integrator4 : Integrator  InitialCondition=zeros(3,1)
  Interpreted MATLAB Function{,20..24} (6 alike) : MATLABFcn  MATLABFcn=cal_frac_squ(u(1:3),u(4),u(5))
  Mux{19..24} (6 alike) : Mux  Inputs=3
  Product : Product
  Product1 : Product
  cal differentiator : MATLAB Function  TreatAsAtomicUnit=on
  cal sig : MATLAB Function  TreatAsAtomicUnit=on
  cal sig1 : MATLAB Function  TreatAsAtomicUnit=on
  cal sig2 : MATLAB Function  TreatAsAtomicUnit=on
  cal sig3 : MATLAB Function  TreatAsAtomicUnit=on
  cal sig4 : MATLAB Function  TreatAsAtomicUnit=on
  cal sig5 : MATLAB Function  TreatAsAtomicUnit=on
  choose sigma_bar_w : MATLAB Function  TreatAsAtomicUnit=on
  sigma_bar_w_tilt : Scope  NumInputPorts=3
  trans to column20 : MATLAB Function  TreatAsAtomicUnit=on
  trans to column21 : MATLAB Function  TreatAsAtomicUnit=on
  trans to column22 : MATLAB Function  TreatAsAtomicUnit=on
  trans to column23 : MATLAB Function  TreatAsAtomicUnit=on
  trans to column24 : MATLAB Function  TreatAsAtomicUnit=on
  trans to column25 : MATLAB Function  TreatAsAtomicUnit=on
  Out1 : Outport
  Out2 : Outport  Port=2
  Out3 : Outport  Port=3
  wires:
  Abs/1 -> Mux22/1
  [sigma_bar_w_tilt] -> cal sig/2(y)
  cal sig1/1(z) -> [sigma_bar_w_sig_2]
  [d2_sigma_bar_w_hat] -> cal differentiator/12(d2_sigma_bar_v_hat)
  trans to column23/1(y) -> [sigma_bar_w_tilt_squ_3]
  Add/1 -> Mux21/2
  Demux2/1 -> sigma_bar_w_tilt/1
  [sigma_bar_w_tilt] -> cal sig4/2(y)
  Product1/1 -> Add2/2
  Add2/1 -> Mux19/2
  [d_sigma_bar_w_hat] -> cal differentiator/11("d_sigma_bar_v_hat ")
  [sigma_bar_w_sig_3] -> cal differentiator/7(sigma_bar_v_sig_3)
  trans to column24/1(y) -> [sigma_bar_w_tilt_squ_4]
  Constant107/1 -> Mux21/3
  [sigma_bar_w_sig_5] -> cal differentiator/9(sigma_bar_v_sig_5)
  Constant97/1 -> Mux22/3
  cal sig/1(z) -> [sigma_bar_w_sig_1]
  trans to column22/1(y) -> [sigma_bar_w_tilt_squ_1]
  [sigma_bar_w_tilt_squ_3] -> cal sig2/1(x)
  [sigma_bar_w_tilt] -> Abs3/1
  Interpreted MATLAB Function24/1 -> trans to column25/1(x)
  [sigma_bar_w_sig_1] -> cal differentiator/5(sigma_bar_v_sig_1)
  cal differentiator/1(d_sigma_bar_v_hat) -> Integrator2/1
  Constant110/1 -> Mux24/3
  cal sig5/1(z) -> [sigma_bar_w_sig_5]
  [sigma_bar_w_tilt] -> Abs4/1
  Demux2/3 -> sigma_bar_w_tilt/3
  cal sig2/1(z) -> [sigma_bar_w_sig_3]
  Constant112/1 -> Product/1
  Constant/1 -> Mux22/2
  cal differentiator/3(d_d2sigma_bar_v_hat) -> Integrator4/1
  Abs3/1 -> Mux24/1
  trans to column21/1(y) -> [sigma_bar_w_tilt_squ_2]
  Constant99/1 -> Add2/1
  Constant103/1 -> cal differentiator/1(c1)
  Mux19/1 -> Interpreted MATLAB Function24/1
  [sigma_bar_w_tilt_squ_6] -> cal sig3/1(x)
  Constant106/1 -> cal differentiator/3(c3)
  [sigma_bar_w_tilt] -> Abs2/1
  [sigma_bar_w_tilt_squ_2] -> cal sig1/1(x)
  Constant162/1 -> Product/2
  Product/1 -> Add1/2
  [sigma_bar_w_sig_4] -> cal differentiator/8(sigma_bar_v_sig_4)
  [sigma_bar_w_hat] -> Add3/1
  Constant102/1 -> Mux20/2
  Add3/1 -> Demux2/1, [sigma_bar_w_tilt]
  cal differentiator/2(d_dsigma_bar_v_hat) -> Integrator3/1
  [sigma_bar_w_tilt] -> Abs5/1
  [sigma_bar_w_tilt] -> cal sig2/2(y)
  [sigma_bar_w_sig_6] -> cal differentiator/10(sigma_bar_v_sig_6)
  trans to column20/1(y) -> [sigma_bar_w_tilt_squ_5]
  Constant104/1 -> cal differentiator/2(c2)
  Constant101/1 -> Mux20/3
  Mux22/1 -> Interpreted MATLAB Function/1
  Constant163/1 -> Product1/2
  Abs2/1 -> Mux23/1
  Interpreted MATLAB Function21/1 -> trans to column21/1(x)
  Interpreted MATLAB Function23/1 -> trans to column24/1(x)
  Mux23/1 -> Interpreted MATLAB Function22/1
  cal sig3/1(z) -> [sigma_bar_w_sig_6]
  Abs4/1 -> Mux19/1
  trans to column25/1(y) -> [sigma_bar_w_tilt_squ_6]
  Constant113/1 -> cal differentiator/4(chi_t)
  choose sigma_bar_w/1(y) -> Add3/2
  Interpreted MATLAB Function/1 -> trans to column22/1(x)
  Interpreted MATLAB Function20/1 -> trans to column20/1(x)
  Constant108/1 -> Mux23/3
  [sigma_bar_w_sig_2] -> cal differentiator/6(sigma_bar_v_sig_2)
  [sigma_bar_w_tilt] -> cal sig1/2(y)
  [sigma_bar_w_tilt_squ_1] -> cal sig/1(x)
  Constant100/1 -> Product1/1
  Abs1/1 -> Mux21/1
  Demux2/2 -> sigma_bar_w_tilt/2
  Integrator4/1 -> [d2_sigma_bar_w_hat], Out3/1
  [sigma_bar_w_tilt_squ_4] -> cal sig4/1(x)
  Abs5/1 -> Mux20/1
  Constant98/1 -> Mux19/3
  Constant111/1 -> Add1/1
  [sigma_bar_w_tilt] -> cal sig5/2(y)
  Constant109/1 -> Mux23/2
  [sigma_bar_w_tilt] -> Abs/1
  Mux24/1 -> Interpreted MATLAB Function23/1
  [sigma_bar_w_tilt] -> Abs1/1
  [sigma_bar_w_tilt_squ_5] -> cal sig5/1(x)
  Add1/1 -> Mux24/2
  cal sig4/1(z) -> [sigma_bar_w_sig_4]
  Constant161/1 -> Add/2
  [sigma_bar_w_tilt] -> cal sig3/2(y)
  Mux21/1 -> Interpreted MATLAB Function21/1
  Interpreted MATLAB Function22/1 -> trans to column23/1(x)
  Mux20/1 -> Interpreted MATLAB Function20/1
  x/1 -> choose sigma_bar_w/1(x)
  Constant105/1 -> Add/1
  Integrator2/1 -> [sigma_bar_w_hat], Out1/1
  Integrator3/1 -> [d_sigma_bar_w_hat], Out2/1

== matlab function sim_tcst_2024_att_ctrl/trans to column30 ==
  data: x input; y output
function y = fcn(x)
y = x(:);

== matlab function sim_tcst_2024_att_ctrl/trans to column31 ==
  data: x input; y output
function y = fcn(x)
y = x(:);

== matlab function sim_tcst_2024_att_ctrl/trans to column32 ==
  data: x input; y output
function y = fcn(x)
y = x(:);

== matlab function sim_tcst_2024_att_ctrl/trans to column33 ==
  data: x input; y output
function y = fcn(x)
y = x(:);

== matlab function sim_tcst_2024_att_ctrl/trans to column34 ==
  data: x input; y output
function y = fcn(x)
y = x(:);

== matlab function sim_tcst_2024_att_ctrl/leader control input ==
  data: t input; u0 output; T1 input; T2 input; R0 input; R1 input; Rx2 input; Ry2 input; Rz2 input
function u0  = fcn(t, T1, T2, R0, R1, Rx2, Ry2, Rz2)
%%%% 给出领导者参考加速度控制输入
u0 = zeros(3, 1);

if t <= ( T1 + 1e-05 )
    u0(1, 1) = - ( 4 * pi * sin( ( 2 * pi * ( t - 0 ) ) / ( 0 - T1 ) ) * ( R0 - R1 ) ) / ( ( 0 - T1 ) ^ 2 ) ...
                        - ( 4 * ( pi ^ 2 ) * cos( ( 2 * pi * ( t - 0 ) ) / ( 0 - T1 ) ) ...
                        * ( R0 + ( ( R0 - R1 ) * ( t - 0 ) ) / ( 0 - T1 ) ) ) / ( ( 0 - T1 ) ^ 2 );
    u0(2, 1) = ( 4 * pi * cos( ( 2 * pi * ( t - 0 ) ) / ( 0 - T1 ) ) * ( R0 - R1 ) ) / ( ( 0 - T1 ) ^ 2 ) ...
                        - ( 4 * ( pi ^ 2 ) * sin( ( 2 * pi * ( t - 0 ) ) / ( 0 - T1 ) ) ...
                        * ( R0 + ( ( R0 - R1 ) * ( t - 0 ) ) / ( 0 - T1 ) ) ) / ( ( 0 - T1 ) ^ 2 );
    u0(3, 1) = 0;
else
    u0(1, 1) = ( 4 * Rx2 * ( pi ^ 2 ) * cos( ( 2 * pi * ( t - T1 ) ) / ( T1 - T2 ) ) ) / ( ( T1 - T2 ) ^ 2 );
    u0(2, 1) = - ( 16 * Ry2 * ( pi ^ 2 ) * sin( ( 4 * pi * ( t - T1 ) ) / ( T1 - T2 ) ) ) / ( ( T1 - T2 ) ^ 2 );
    u0(3, 1) = ( 16 * Rz2 * ( pi ^ 2 ) * sin( ( 4 * pi * ( t - T1 ) ) / ( T1 - T2 ) ) ) / ( ( T1 - T2 ) ^ 2 );
end

== matlab function sim_tcst_2024_att_ctrl/combine duihat d2uihat ==
  data: d_ui_hat_node_1 input; duihat_vec output; d2uihat_vec output; d_ui_hat_node_2 input; d_ui_hat_node_3 input; d_ui_hat_node_4 input; d_ui_hat_node_5 input; d2_ui_hat_node_1 input; d2_ui_hat_node_2 input; d2_ui_hat_node_3 input; d2_ui_hat_node_4 input; d2_ui_hat_node_5 input
function [duihat_vec, d2uihat_vec] = fcn(d_ui_hat_node_1, d_ui_hat_node_2, d_ui_hat_node_3, d_ui_hat_node_4, d_ui_hat_node_5, ...
                                                                            d2_ui_hat_node_1, d2_ui_hat_node_2, d2_ui_hat_node_3, d2_ui_hat_node_4, d2_ui_hat_node_5)

duihat_vec = [d_ui_hat_node_1(:), d_ui_hat_node_2(:), d_ui_hat_node_3(:), d_ui_hat_node_4(:), d_ui_hat_node_5(:)];
d2uihat_vec = [d2_ui_hat_node_1(:), d2_ui_hat_node_2(:), d2_ui_hat_node_3(:), d2_ui_hat_node_4(:), d2_ui_hat_node_5(:)];

== matlab function sim_tcst_2024_att_ctrl/cal wci dwci agent 1 ==
  data: ui_vec input; wci output; duihat_vec input; d2uihat_vec input; Rci_mat input; dwci output
function [wci, dwci] = fcn(ui_vec, duihat_vec, d2uihat_vec, Rci_mat)
%%%% 计算姿态角速率指令及其导数

iiuav = 1;
ui = ui_vec(:,iiuav);
duihat = duihat_vec(:,iiuav);
d2uihat = d2uihat_vec(:,iiuav);
Rci = Rci_mat(:,:,iiuav);

ee1 = [1;0;0];
ee2 = [0;1;0];
ee3 = [0;0;1];
RciE3 = ui / norm(ui,2);
PiMat = eye(3,3) - ee3*(ee3');
dRciE3 = (1 / norm(ui,2))*Rci*PiMat*(Rci')*duihat;
Themat = [-RciE3(2)/(1+RciE3(3)),         -RciE3(1)/(1+RciE3(3)),       (RciE3(1)*RciE3(2))/((1+RciE3(3))^2); ...
                   2*RciE3(1)/(1+RciE3(3)),                0,                               1 - (RciE3(1)^2)/((1+RciE3(3))^2); ...
                               0                                       -1                                                        0                                   ];
wcxe3 = (1 / norm(ui,2))*PiMat*(Rci')*duihat;
wcxe2 = (1 / norm(ui,2))*(Rci')*Themat*Rci*PiMat*(Rci')*duihat;
wci = [-wcxe3(2); wcxe3(1); -wcxe2(1)];

TempMat1 = [0,                           -1/(1+RciE3(3)),                   (RciE3(2))/((1+RciE3(3))^2); ...
                       2/(1+RciE3(3)),                0,                               (-2*RciE3(1))/((1+RciE3(3))^2); ...
                       0,                                     0,                                                   0                             ];
TempMat2 = [-1/(1+RciE3(3)),              0,                               (RciE3(1))/((1+RciE3(3))^2); ...
                       0,                                     0,                                                   0                      ; ...
                       0,                                     0,                                                   0                             ];
TempMat3 = [(RciE3(2))/((1+RciE3(3))^2),                 (RciE3(1))/((1+RciE3(3))^2),       (-2*RciE3(1)*RciE3(2))/((1+RciE3(3))^3); ...
                       (-2*RciE3(1))/((1+RciE3(3))^2),                             0,                               (2*(RciE3(1)^2))/((1+RciE3(3))^3); ...
                        0,                                                                          0,                                                   0                             ];
dTheMat = TempMat1*dRciE3*(ee1') + TempMat2*dRciE3*(ee2') + TempMat3*dRciE3*(ee3');
wcix = cal_askew_mat(wci);
dRciT = -wcix*(Rci');
dwcxe3 = (1 / norm(ui,2))*PiMat*(dRciT*duihat+(Rci')*(d2uihat-(((ui')*duihat)/(norm(ui,2)^2))*duihat));
dwcxe2 = (1 / norm(ui,2))*((dRciT*Themat+(Rci')*dTheMat) ...
                *(Rci*PiMat*(Rci'))*duihat + (Rci')*Themat*(Rci*PiMat*(Rci'))*(d2uihat-(((ui')*duihat)/(norm(ui,2)^2))*duihat));
dwci = [-dwcxe3(2);  dwcxe3(1);  -dwcxe2(1)];

== matlab function sim_tcst_2024_att_ctrl/cal wci dwci agent 2 ==
  data: ui_vec input; wci output; duihat_vec input; d2uihat_vec input; Rci_mat input; dwci output
function [wci, dwci] = fcn(ui_vec, duihat_vec, d2uihat_vec, Rci_mat)
%%%% 计算姿态角速率指令及其导数

iiuav = 2;
ui = ui_vec(:,iiuav);
duihat = duihat_vec(:,iiuav);
d2uihat = d2uihat_vec(:,iiuav);
Rci = Rci_mat(:,:,iiuav);

ee1 = [1;0;0];
ee2 = [0;1;0];
ee3 = [0;0;1];
RciE3 = ui / norm(ui,2);
PiMat = eye(3,3) - ee3*(ee3');
dRciE3 = (1 / norm(ui,2))*Rci*PiMat*(Rci')*duihat;
Themat = [-RciE3(2)/(1+RciE3(3)),         -RciE3(1)/(1+RciE3(3)),       (RciE3(1)*RciE3(2))/((1+RciE3(3))^2); ...
                   2*RciE3(1)/(1+RciE3(3)),                0,                               1 - (RciE3(1)^2)/((1+RciE3(3))^2); ...
                               0                                       -1                                                        0                                   ];
wcxe3 = (1 / norm(ui,2))*PiMat*(Rci')*duihat;
wcxe2 = (1 / norm(ui,2))*(Rci')*Themat*Rci*PiMat*(Rci')*duihat;
wci = [-wcxe3(2); wcxe3(1); -wcxe2(1)];

TempMat1 = [0,                           -1/(1+RciE3(3)),                   (RciE3(2))/((1+RciE3(3))^2); ...
                       2/(1+RciE3(3)),                0,                               (-2*RciE3(1))/((1+RciE3(3))^2); ...
                       0,                                     0,                                                   0                             ];
TempMat2 = [-1/(1+RciE3(3)),              0,                               (RciE3(1))/((1+RciE3(3))^2); ...
                       0,                                     0,                                                   0                      ; ...
                       0,                                     0,                                                   0                             ];
TempMat3 = [(RciE3(2))/((1+RciE3(3))^2),                 (RciE3(1))/((1+RciE3(3))^2),       (-2*RciE3(1)*RciE3(2))/((1+RciE3(3))^3); ...
                       (-2*RciE3(1))/((1+RciE3(3))^2),                             0,                               (2*(RciE3(1)^2))/((1+RciE3(3))^3); ...
                        0,                                                                          0,                                                   0                             ];
dTheMat = TempMat1*dRciE3*(ee1') + TempMat2*dRciE3*(ee2') + TempMat3*dRciE3*(ee3');
wcix = cal_askew_mat(wci);
dRciT = -wcix*(Rci');
dwcxe3 = (1 / norm(ui,2))*PiMat*(dRciT*duihat+(Rci')*(d2uihat-(((ui')*duihat)/(norm(ui,2)^2))*duihat));
dwcxe2 = (1 / norm(ui,2))*((dRciT*Themat+(Rci')*dTheMat) ...
                *(Rci*PiMat*(Rci'))*duihat + (Rci')*Themat*(Rci*PiMat*(Rci'))*(d2uihat-(((ui')*duihat)/(norm(ui,2)^2))*duihat));
dwci = [-dwcxe3(2);  dwcxe3(1);  -dwcxe2(1)];

== matlab function sim_tcst_2024_att_ctrl/cal wci dwci agent 3 ==
  data: ui_vec input; wci output; duihat_vec input; d2uihat_vec input; Rci_mat input; dwci output
function [wci, dwci] = fcn(ui_vec, duihat_vec, d2uihat_vec, Rci_mat)
%%%% 计算姿态角速率指令及其导数

iiuav = 3;
ui = ui_vec(:,iiuav);
duihat = duihat_vec(:,iiuav);
d2uihat = d2uihat_vec(:,iiuav);
Rci = Rci_mat(:,:,iiuav);

ee1 = [1;0;0];
ee2 = [0;1;0];
ee3 = [0;0;1];
RciE3 = ui / norm(ui,2);
PiMat = eye(3,3) - ee3*(ee3');
dRciE3 = (1 / norm(ui,2))*Rci*PiMat*(Rci')*duihat;
Themat = [-RciE3(2)/(1+RciE3(3)),         -RciE3(1)/(1+RciE3(3)),       (RciE3(1)*RciE3(2))/((1+RciE3(3))^2); ...
                   2*RciE3(1)/(1+RciE3(3)),                0,                               1 - (RciE3(1)^2)/((1+RciE3(3))^2); ...
                               0                                       -1                                                        0                                   ];
wcxe3 = (1 / norm(ui,2))*PiMat*(Rci')*duihat;
wcxe2 = (1 / norm(ui,2))*(Rci')*Themat*Rci*PiMat*(Rci')*duihat;
wci = [-wcxe3(2); wcxe3(1); -wcxe2(1)];

TempMat1 = [0,                           -1/(1+RciE3(3)),                   (RciE3(2))/((1+RciE3(3))^2); ...
                       2/(1+RciE3(3)),                0,                               (-2*RciE3(1))/((1+RciE3(3))^2); ...
                       0,                                     0,                                                   0                             ];
TempMat2 = [-1/(1+RciE3(3)),              0,                               (RciE3(1))/((1+RciE3(3))^2); ...
                       0,                                     0,                                                   0                      ; ...
                       0,                                     0,                                                   0                             ];
TempMat3 = [(RciE3(2))/((1+RciE3(3))^2),                 (RciE3(1))/((1+RciE3(3))^2),       (-2*RciE3(1)*RciE3(2))/((1+RciE3(3))^3); ...
                       (-2*RciE3(1))/((1+RciE3(3))^2),                             0,                               (2*(RciE3(1)^2))/((1+RciE3(3))^3); ...
                        0,                                                                          0,                                                   0                             ];
dTheMat = TempMat1*dRciE3*(ee1') + TempMat2*dRciE3*(ee2') + TempMat3*dRciE3*(ee3');
wcix = cal_askew_mat(wci);
dRciT = -wcix*(Rci');
dwcxe3 = (1 / norm(ui,2))*PiMat*(dRciT*duihat+(Rci')*(d2uihat-(((ui')*duihat)/(norm(ui,2)^2))*duihat));
dwcxe2 = (1 / norm(ui,2))*((dRciT*Themat+(Rci')*dTheMat) ...
                *(Rci*PiMat*(Rci'))*duihat + (Rci')*Themat*(Rci*PiMat*(Rci'))*(d2uihat-(((ui')*duihat)/(norm(ui,2)^2))*duihat));
dwci = [-dwcxe3(2);  dwcxe3(1);  -dwcxe2(1)];

== matlab function sim_tcst_2024_att_ctrl/cal wci dwci agent 4 ==
  data: ui_vec input; wci output; duihat_vec input; d2uihat_vec input; Rci_mat input; dwci output
function [wci, dwci] = fcn(ui_vec, duihat_vec, d2uihat_vec, Rci_mat)
%%%% 计算姿态角速率指令及其导数

iiuav = 4;
ui = ui_vec(:,iiuav);
duihat = duihat_vec(:,iiuav);
d2uihat = d2uihat_vec(:,iiuav);
Rci = Rci_mat(:,:,iiuav);

ee1 = [1;0;0];
ee2 = [0;1;0];
ee3 = [0;0;1];
RciE3 = ui / norm(ui,2);
PiMat = eye(3,3) - ee3*(ee3');
dRciE3 = (1 / norm(ui,2))*Rci*PiMat*(Rci')*duihat;
Themat = [-RciE3(2)/(1+RciE3(3)),         -RciE3(1)/(1+RciE3(3)),       (RciE3(1)*RciE3(2))/((1+RciE3(3))^2); ...
                   2*RciE3(1)/(1+RciE3(3)),                0,                               1 - (RciE3(1)^2)/((1+RciE3(3))^2); ...
                               0                                       -1                                                        0                                   ];
wcxe3 = (1 / norm(ui,2))*PiMat*(Rci')*duihat;
wcxe2 = (1 / norm(ui,2))*(Rci')*Themat*Rci*PiMat*(Rci')*duihat;
wci = [-wcxe3(2); wcxe3(1); -wcxe2(1)];

TempMat1 = [0,                           -1/(1+RciE3(3)),                   (RciE3(2))/((1+RciE3(3))^2); ...
                       2/(1+RciE3(3)),                0,                               (-2*RciE3(1))/((1+RciE3(3))^2); ...
                       0,                                     0,                                                   0                             ];
TempMat2 = [-1/(1+RciE3(3)),              0,                               (RciE3(1))/((1+RciE3(3))^2); ...
                       0,                                     0,                                                   0                      ; ...
                       0,                                     0,                                                   0                             ];
TempMat3 = [(RciE3(2))/((1+RciE3(3))^2),                 (RciE3(1))/((1+RciE3(3))^2),       (-2*RciE3(1)*RciE3(2))/((1+RciE3(3))^3); ...
                       (-2*RciE3(1))/((1+RciE3(3))^2),                             0,                               (2*(RciE3(1)^2))/((1+RciE3(3))^3); ...
                        0,                                                                          0,                                                   0                             ];
dTheMat = TempMat1*dRciE3*(ee1') + TempMat2*dRciE3*(ee2') + TempMat3*dRciE3*(ee3');
wcix = cal_askew_mat(wci);
dRciT = -wcix*(Rci');
dwcxe3 = (1 / norm(ui,2))*PiMat*(dRciT*duihat+(Rci')*(d2uihat-(((ui')*duihat)/(norm(ui,2)^2))*duihat));
dwcxe2 = (1 / norm(ui,2))*((dRciT*Themat+(Rci')*dTheMat) ...
                *(Rci*PiMat*(Rci'))*duihat + (Rci')*Themat*(Rci*PiMat*(Rci'))*(d2uihat-(((ui')*duihat)/(norm(ui,2)^2))*duihat));
dwci = [-dwcxe3(2);  dwcxe3(1);  -dwcxe2(1)];

== matlab function sim_tcst_2024_att_ctrl/cal wci dwci agent 5 ==
  data: ui_vec input; wci output; duihat_vec input; d2uihat_vec input; Rci_mat input; dwci output
function [wci, dwci] = fcn(ui_vec, duihat_vec, d2uihat_vec, Rci_mat)
%%%% 计算姿态角速率指令及其导数

iiuav = 5;
ui = ui_vec(:,iiuav);
duihat = duihat_vec(:,iiuav);
d2uihat = d2uihat_vec(:,iiuav);
Rci = Rci_mat(:,:,iiuav);

ee1 = [1;0;0];
ee2 = [0;1;0];
ee3 = [0;0;1];
RciE3 = ui / norm(ui,2);
PiMat = eye(3,3) - ee3*(ee3');
dRciE3 = (1 / norm(ui,2))*Rci*PiMat*(Rci')*duihat;
Themat = [-RciE3(2)/(1+RciE3(3)),         -RciE3(1)/(1+RciE3(3)),       (RciE3(1)*RciE3(2))/((1+RciE3(3))^2); ...
                   2*RciE3(1)/(1+RciE3(3)),                0,                               1 - (RciE3(1)^2)/((1+RciE3(3))^2); ...
                               0                                       -1                                                        0                                   ];
wcxe3 = (1 / norm(ui,2))*PiMat*(Rci')*duihat;
wcxe2 = (1 / norm(ui,2))*(Rci')*Themat*Rci*PiMat*(Rci')*duihat;
wci = [-wcxe3(2); wcxe3(1); -wcxe2(1)];

TempMat1 = [0,                           -1/(1+RciE3(3)),                   (RciE3(2))/((1+RciE3(3))^2); ...
                       2/(1+RciE3(3)),                0,                               (-2*RciE3(1))/((1+RciE3(3))^2); ...
                       0,                                     0,                                                   0                             ];
TempMat2 = [-1/(1+RciE3(3)),              0,                               (RciE3(1))/((1+RciE3(3))^2); ...
                       0,                                     0,                                                   0                      ; ...
                       0,                                     0,                                                   0                             ];
TempMat3 = [(RciE3(2))/((1+RciE3(3))^2),                 (RciE3(1))/((1+RciE3(3))^2),       (-2*RciE3(1)*RciE3(2))/((1+RciE3(3))^3); ...
                       (-2*RciE3(1))/((1+RciE3(3))^2),                             0,                               (2*(RciE3(1)^2))/((1+RciE3(3))^3); ...
                        0,                                                                          0,                                                   0                             ];
dTheMat = TempMat1*dRciE3*(ee1') + TempMat2*dRciE3*(ee2') + TempMat3*dRciE3*(ee3');
wcix = cal_askew_mat(wci);
dRciT = -wcix*(Rci');
dwcxe3 = (1 / norm(ui,2))*PiMat*(dRciT*duihat+(Rci')*(d2uihat-(((ui')*duihat)/(norm(ui,2)^2))*duihat));
dwcxe2 = (1 / norm(ui,2))*((dRciT*Themat+(Rci')*dTheMat) ...
                *(Rci*PiMat*(Rci'))*duihat + (Rci')*Themat*(Rci*PiMat*(Rci'))*(d2uihat-(((ui')*duihat)/(norm(ui,2)^2))*duihat));
dwci = [-dwcxe3(2);  dwcxe3(1);  -dwcxe2(1)];

== matlab function sim_tcst_2024_att_ctrl/depart err_Ri_bar 3 ==
  data: y output; x input
function y = fcn(x)
y = x(:,3);

end

== matlab function sim_tcst_2024_att_ctrl/depart err_Ri_bar 4 ==
  data: y output; x input
function y = fcn(x)
y = x(:,4);

end
